simulink model "untitled"  (Simulink 8.8)
settings: Solver=ode3  StartTime=0.0  StopTime=0.092  FixedStep=10^(-6)  RelTol=1e-3  EnableMultiTasking=on
libraries: simulink x2
settings Model: Creator=student  LastModifiedBy=Admin
settings OptimizationCC: ExpressionDepthLimit=2147483647  InitFltsAndDblsToZero=on
settings DebuggingCC: SaveWithParameterizedLinksMsg=none  SolverPrmCheckMsg=warning
settings GRTTargetCC: TargetFcnLib=ansi_tfl_tmw.mat  GeneratePreprocessorConditionals=Use local settings

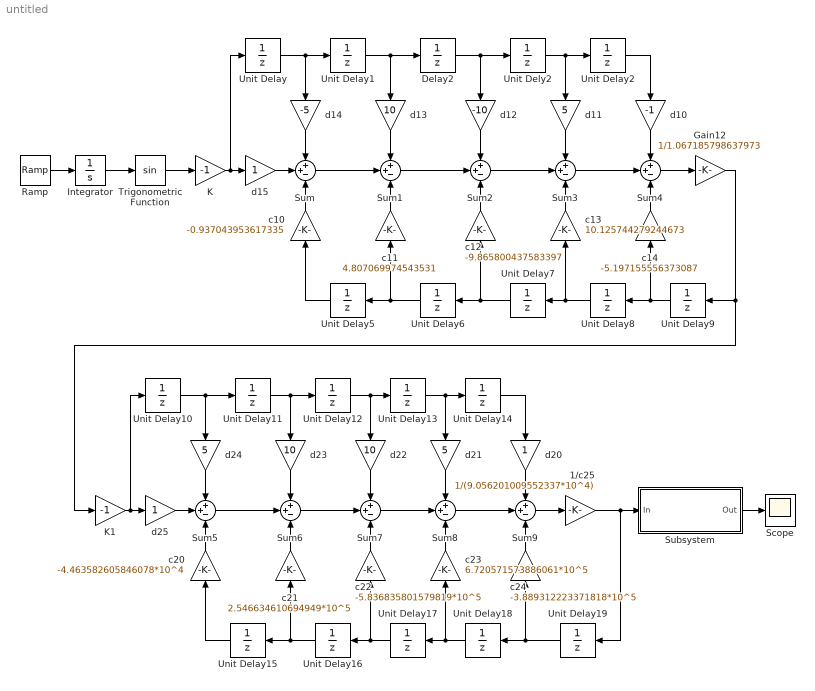
== system untitled ==
  1/c25 : Gain  Gain=1/(9.056201009552337*10^4)
  Delay2 : UnitDelay  SampleTime=10^(-6)
  Gain12 : Gain  Gain=1/1.067185798637973
  Integrator : Integrator
  K : Gain  Gain=-1
  K1 : Gain  Gain=-1
  Ramp : simulink/Sources/Ramp  slope=1.191227230625727*10^7  start=0  X0=0
  Scope : Scope
  Subsystem : Subsystem
  Sum{,1..9} (10 alike) : Sum  Inputs=++-
  Trigonometric Function : Trigonometry
  Unit Delay{,1..2,5..19} (18 alike) : UnitDelay  SampleTime=10^(-6)
  Unit Dely2 : UnitDelay  SampleTime=10^(-6)
  c10 : Gain  Gain=-0.937043953617335
  c11 : Gain  Gain=4.807069974543531
  c12 : Gain  Gain=-9.865800437583397
  c13 : Gain  Gain=10.125744279244673
  c14 : Gain  Gain=-5.197155556373087
  c20 : Gain  Gain=-4.463582605846078*10^4
  c21 : Gain  Gain=2.546634610694949*10^5
  c22 : Gain  Gain=-5.836835801579819*10^5
  c23 : Gain  Gain=6.720571573886061*10^5
  c24 : Gain  Gain=-3.889312223371818*10^5
  d10 : Gain  Gain=-1
  d11 : Gain  Gain=5
  d12 : Gain  Gain=-10
  d13 : Gain  Gain=10
  d14 : Gain  Gain=-5
  d15 : Gain
  d20 : Gain
  d21 : Gain  Gain=5
  d22 : Gain  Gain=10
  d23 : Gain  Gain=10
  d24 : Gain  Gain=5
  d25 : Gain
  wires:
  Ramp/1 -> Integrator/1
  Integrator/1 -> Trigonometric Function/1
  Trigonometric Function/1 -> K/1
  K/1 -> d15/1, Unit Delay/1
  d15/1 -> Sum/2
  Sum/1 -> Sum1/2
  Sum1/1 -> Sum2/2
  Sum2/1 -> Sum3/2
  Sum3/1 -> Sum4/2
  Unit Delay/1 -> Unit Delay1/1, d14/1
  Unit Delay1/1 -> Delay2/1, d13/1
  Delay2/1 -> Unit Dely2/1, d12/1
  Unit Dely2/1 -> Unit Delay2/1, d11/1
  Unit Delay2/1 -> d10/1
  d11/1 -> Sum3/1
  d10/1 -> Sum4/1
  d12/1 -> Sum2/1
  d13/1 -> Sum1/1
  d14/1 -> Sum/1
  c10/1 -> Sum/3
  c11/1 -> Sum1/3
  c12/1 -> Sum2/3
  c13/1 -> Sum3/3
  c14/1 -> Sum4/3
  Unit Delay9/1 -> Unit Delay8/1, c14/1
  Unit Delay8/1 -> Unit Delay7/1, c13/1
  Unit Delay7/1 -> Unit Delay6/1, c12/1
  Unit Delay6/1 -> Unit Delay5/1, c11/1
  Unit Delay5/1 -> c10/1
  Sum4/1 -> Gain12/1
  Gain12/1 -> Unit Delay9/1, K1/1
  K1/1 -> d25/1, Unit Delay10/1
  d25/1 -> Sum5/2
  Sum5/1 -> Sum6/2
  Sum6/1 -> Sum7/2
  Sum7/1 -> Sum8/2
  Sum8/1 -> Sum9/2
  Unit Delay10/1 -> Unit Delay11/1, d24/1
  Unit Delay11/1 -> Unit Delay12/1, d23/1
  Unit Delay12/1 -> Unit Delay13/1, d22/1
  Unit Delay13/1 -> Unit Delay14/1, d21/1
  Unit Delay14/1 -> d20/1
  d21/1 -> Sum8/1
  d20/1 -> Sum9/1
  d22/1 -> Sum7/1
  d23/1 -> Sum6/1
  d24/1 -> Sum5/1
  c20/1 -> Sum5/3
  c21/1 -> Sum6/3
  c22/1 -> Sum7/3
  c23/1 -> Sum8/3
  c24/1 -> Sum9/3
  Unit Delay19/1 -> c24/1, Unit Delay18/1
  Unit Delay18/1 -> Unit Delay17/1, c23/1
  Unit Delay17/1 -> Unit Delay16/1, c22/1
  Unit Delay16/1 -> Unit Delay15/1, c21/1
  Unit Delay15/1 -> c20/1
  Sum9/1 -> 1/c25/1
  1/c25/1 -> Unit Delay19/1, Subsystem/1(In)
  Subsystem/1(Out) -> Scope/1

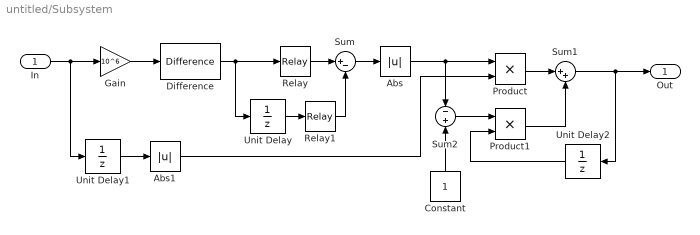
== system untitled/Subsystem ==
  In : Inport
  Abs : Abs
  Abs1 : Abs
  Constant : Constant
  Difference : simulink/Discrete/Difference  ICPrevInput=0.0  InputProcessing=Inherited  OutMin=[]  OutMax=[]  OutDataType=sfix(16)  OutScaling=2^-10  DoSatur=off
  Gain : Gain  Gain=10^6
  Product : Product  RndMeth=Zero
  Product1 : Product  RndMeth=Zero
  Relay : Relay  OnSwitchValue=0  OffSwitchValue=0
  Relay1 : Relay  OnSwitchValue=0  OffSwitchValue=0
  Sum : Sum  Inputs=|+-
  Sum1 : Sum  Inputs=|++
  Sum2 : Sum  Inputs=-|+
  Unit Delay : UnitDelay  SampleTime=10^(-6)
  Unit Delay1 : UnitDelay  SampleTime=10^(-6)
  Unit Delay2 : UnitDelay  SampleTime=10^(-6)
  Out : Outport
  wires:
  In/1 -> Gain/1, Unit Delay1/1
  Gain/1 -> Difference/1
  Unit Delay/1 -> Relay1/1
  Difference/1 -> Relay/1, Unit Delay/1
  Relay/1 -> Sum/1
  Relay1/1 -> Sum/2
  Sum/1 -> Abs/1
  Abs/1 -> Product/1, Sum2/1
  Unit Delay1/1 -> Abs1/1
  Product/1 -> Sum1/1
  Abs1/1 -> Product/2
  Constant/1 -> Sum2/2
  Sum2/1 -> Product1/1
  Unit Delay2/1 -> Product1/2
  Sum1/1 -> Out/1, Unit Delay2/1
  Product1/1 -> Sum1/2
